simulink model "Model_AC_TES_Double_Coil"  (R2025b)
settings: Solver=VariableStepAuto  StartTime=0.0  StopTime=3600*9  RelTol=1e-3
model workspace (MAT data in the model file):
  COP = 3.9
  Delayfan = [30 1]
  P1 = 1.05
  P2 = 1.91
  P3 = 1.91
  P4 = 1.05
  Q_Cond = 4.361
  Q_Evap = 3.471
  T1 = 12
  T2 = 37.72
  T3 = 29.61
  T4 = 7.9
  T_Enviroment_C = 27.5
  T_Room_int_C = 28.6
  T_Tank_int_c = 30
  Wall_h_in = 12
  Wall_h_out = 38
  h1 = 522.3
  h2 = 528.6
  h3 = 253.4
  h4 = 253.4
  m_dot = 0.014
libraries: fl_lib x102, nesl_utility x62, SimscapeFluids_lib x31
(part 3 of 3)

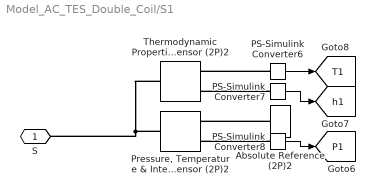
== system Model_AC_TES_Double_Coil/S1 ==
  Absolute Reference (2P)2 : fl_lib/Two-Phase Fluid/Elements/Absolute Reference (2P)
  PS-Simulink Converter6 : nesl_utility/PS-Simulink Converter  PhysicalDomain=network_engine_domain  SubClassName=ps_output  LeftPortType=input  RightPortType=output  PseudoPeriodic=off  Frequencies=[]  VectorFormat=inherit  Unit=degC  AffineConversion=on
  PS-Simulink Converter7 : nesl_utility/PS-Simulink Converter  PhysicalDomain=network_engine_domain  SubClassName=ps_output  LeftPortType=input  RightPortType=output  PseudoPeriodic=off  Frequencies=[]  VectorFormat=inherit  Unit=inherit  AffineConversion=off
  PS-Simulink Converter8 : nesl_utility/PS-Simulink Converter  PhysicalDomain=network_engine_domain  SubClassName=ps_output  LeftPortType=input  RightPortType=output  PseudoPeriodic=off  Frequencies=[]  VectorFormat=inherit  Unit=inherit  AffineConversion=off
  "Pressure, Temperature & Internal Energy Sensor (2P)2" : fl_lib/Two-Phase Fluid/Sensors/Pressure, Temperature & Internal Energy Sensor (2P)  reference=foundation.enum.MeasurementReference.difference  pressure=true  pressure_spec=foundation.enum.PressureMeasementSpec.Absolute  temperature=false  internal_energy=false
      settings: InternalSimscapePortConfiguration="{\"Bottom\":[],\"Left\":[{\"id\":\"A\",\"label\":\"A\",\"type\":\"foundation.two_phase_fluid.two_phase_fluid\"}],\"Right\":[{\"id\":\"B\",\"label\":\"B\",\"type\":\"foundation.two_phase_fluid.two_phase_fluid\"},{\"id\":\"P\",\"label\":\"P\",\"type\":\"output\"}],\"Top\":[]}"
  Thermodynamic Properties Sensor (2P)2 : fl_lib/Two-Phase Fluid/Sensors/Thermodynamic Properties Sensor (2P)  temperature=true  enthalpy=true  density=false  specific_volume=false  entropy=false
      settings: InternalSimscapePortConfiguration="{\"Bottom\":[],\"Left\":[{\"id\":\"A\",\"label\":\"A\",\"type\":\"foundation.two_phase_fluid.two_phase_fluid\"}],\"Right\":[{\"id\":\"T\",\"label\":\"T\",\"type\":\"output\"},{\"id\":\"H\",\"label\":\"h\",\"type\":\"output\"}],\"Top\":[]}"
  S : PMIOPort  Side=Left
  tag scope: P1=global, T1=global, h1=global
  wires:
  PS-Simulink Converter8/1 -> [P1]
  PS-Simulink Converter7/1 -> [h1]
  PS-Simulink Converter6/1 -> [T1]
  connections:
  Thermodynamic Properties Sensor (2P)2/LConn1 -- "Pressure, Temperature & Internal Energy Sensor (2P)2"/LConn1 -- S/RConn1
  Absolute Reference (2P)2/LConn1 -- "Pressure, Temperature & Internal Energy Sensor (2P)2"/RConn1
  PS-Simulink Converter7/LConn1 -- Thermodynamic Properties Sensor (2P)2/RConn2
  PS-Simulink Converter8/LConn1 -- "Pressure, Temperature & Internal Energy Sensor (2P)2"/RConn2
  PS-Simulink Converter6/LConn1 -- Thermodynamic Properties Sensor (2P)2/RConn1

== system Model_AC_TES_Double_Coil/S2 ==
  Absolute Reference (2P) : fl_lib/Two-Phase Fluid/Elements/Absolute Reference (2P)
  PS-Simulink Converter : nesl_utility/PS-Simulink Converter  PhysicalDomain=network_engine_domain  SubClassName=ps_output  LeftPortType=input  RightPortType=output  PseudoPeriodic=off  Frequencies=[]  VectorFormat=inherit  Unit=degC  AffineConversion=on
  PS-Simulink Converter1 : nesl_utility/PS-Simulink Converter  PhysicalDomain=network_engine_domain  SubClassName=ps_output  LeftPortType=input  RightPortType=output  PseudoPeriodic=off  Frequencies=[]  VectorFormat=inherit  Unit=inherit  AffineConversion=off
  PS-Simulink Converter2 : nesl_utility/PS-Simulink Converter  PhysicalDomain=network_engine_domain  SubClassName=ps_output  LeftPortType=input  RightPortType=output  PseudoPeriodic=off  Frequencies=[]  VectorFormat=inherit  Unit=inherit  AffineConversion=off
  "Pressure, Temperature & Internal Energy Sensor (2P)" : fl_lib/Two-Phase Fluid/Sensors/Pressure, Temperature & Internal Energy Sensor (2P)  reference=foundation.enum.MeasurementReference.difference  pressure=true  pressure_spec=foundation.enum.PressureMeasementSpec.Absolute  temperature=false  internal_energy=false
      settings: InternalSimscapePortConfiguration="{\"Bottom\":[],\"Left\":[{\"id\":\"A\",\"label\":\"A\",\"type\":\"foundation.two_phase_fluid.two_phase_fluid\"}],\"Right\":[{\"id\":\"B\",\"label\":\"B\",\"type\":\"foundation.two_phase_fluid.two_phase_fluid\"},{\"id\":\"P\",\"label\":\"P\",\"type\":\"output\"}],\"Top\":[]}"
  Thermodynamic Properties Sensor (2P) : fl_lib/Two-Phase Fluid/Sensors/Thermodynamic Properties Sensor (2P)  temperature=true  enthalpy=true  density=false  specific_volume=false  entropy=false
      settings: InternalSimscapePortConfiguration="{\"Bottom\":[],\"Left\":[{\"id\":\"A\",\"label\":\"A\",\"type\":\"foundation.two_phase_fluid.two_phase_fluid\"}],\"Right\":[{\"id\":\"T\",\"label\":\"T\",\"type\":\"output\"},{\"id\":\"H\",\"label\":\"h\",\"type\":\"output\"}],\"Top\":[]}"
  S : PMIOPort  Side=Left
  tag scope: P2=global, T2=global, h2=global
  wires:
  PS-Simulink Converter1/1 -> [h2]
  PS-Simulink Converter/1 -> [T2]
  PS-Simulink Converter2/1 -> [P2]
  connections:
  PS-Simulink Converter2/LConn1 -- "Pressure, Temperature & Internal Energy Sensor (2P)"/RConn2
  PS-Simulink Converter/LConn1 -- Thermodynamic Properties Sensor (2P)/RConn1
  Thermodynamic Properties Sensor (2P)/LConn1 -- "Pressure, Temperature & Internal Energy Sensor (2P)"/LConn1 -- S/RConn1
  Absolute Reference (2P)/LConn1 -- "Pressure, Temperature & Internal Energy Sensor (2P)"/RConn1
  PS-Simulink Converter1/LConn1 -- Thermodynamic Properties Sensor (2P)/RConn2

== system Model_AC_TES_Double_Coil/S3 ==
  Absolute Reference (2P)1 : fl_lib/Two-Phase Fluid/Elements/Absolute Reference (2P)
  PS-Simulink Converter3 : nesl_utility/PS-Simulink Converter  PhysicalDomain=network_engine_domain  SubClassName=ps_output  LeftPortType=input  RightPortType=output  PseudoPeriodic=off  Frequencies=[]  VectorFormat=inherit  Unit=degC  AffineConversion=on
  PS-Simulink Converter4 : nesl_utility/PS-Simulink Converter  PhysicalDomain=network_engine_domain  SubClassName=ps_output  LeftPortType=input  RightPortType=output  PseudoPeriodic=off  Frequencies=[]  VectorFormat=inherit  Unit=inherit  AffineConversion=off
  PS-Simulink Converter5 : nesl_utility/PS-Simulink Converter  PhysicalDomain=network_engine_domain  SubClassName=ps_output  LeftPortType=input  RightPortType=output  PseudoPeriodic=off  Frequencies=[]  VectorFormat=inherit  Unit=inherit  AffineConversion=off
  "Pressure, Temperature & Internal Energy Sensor (2P)1" : fl_lib/Two-Phase Fluid/Sensors/Pressure, Temperature & Internal Energy Sensor (2P)  reference=foundation.enum.MeasurementReference.difference  pressure=true  pressure_spec=foundation.enum.PressureMeasementSpec.Absolute  temperature=false  internal_energy=false
      settings: InternalSimscapePortConfiguration="{\"Bottom\":[],\"Left\":[{\"id\":\"A\",\"label\":\"A\",\"type\":\"foundation.two_phase_fluid.two_phase_fluid\"}],\"Right\":[{\"id\":\"B\",\"label\":\"B\",\"type\":\"foundation.two_phase_fluid.two_phase_fluid\"},{\"id\":\"P\",\"label\":\"P\",\"type\":\"output\"}],\"Top\":[]}"
  Thermodynamic Properties Sensor (2P)1 : fl_lib/Two-Phase Fluid/Sensors/Thermodynamic Properties Sensor (2P)  temperature=true  enthalpy=true  density=false  specific_volume=false  entropy=false
      settings: InternalSimscapePortConfiguration="{\"Bottom\":[],\"Left\":[{\"id\":\"A\",\"label\":\"A\",\"type\":\"foundation.two_phase_fluid.two_phase_fluid\"}],\"Right\":[{\"id\":\"T\",\"label\":\"T\",\"type\":\"output\"},{\"id\":\"H\",\"label\":\"h\",\"type\":\"output\"}],\"Top\":[]}"
  S : PMIOPort  Side=Left
  tag scope: P3=global, T3=global, h3=global
  wires:
  PS-Simulink Converter4/1 -> [h3]
  PS-Simulink Converter3/1 -> [T3]
  PS-Simulink Converter5/1 -> [P3]
  connections:
  Absolute Reference (2P)1/LConn1 -- "Pressure, Temperature & Internal Energy Sensor (2P)1"/RConn1
  PS-Simulink Converter3/LConn1 -- Thermodynamic Properties Sensor (2P)1/RConn1
  PS-Simulink Converter4/LConn1 -- Thermodynamic Properties Sensor (2P)1/RConn2
  Thermodynamic Properties Sensor (2P)1/LConn1 -- "Pressure, Temperature & Internal Energy Sensor (2P)1"/LConn1 -- S/RConn1
  PS-Simulink Converter5/LConn1 -- "Pressure, Temperature & Internal Energy Sensor (2P)1"/RConn2

== system Model_AC_TES_Double_Coil/S4 ==
  Absolute Reference (2P)2 : fl_lib/Two-Phase Fluid/Elements/Absolute Reference (2P)
  PS-Simulink Converter6 : nesl_utility/PS-Simulink Converter  PhysicalDomain=network_engine_domain  SubClassName=ps_output  LeftPortType=input  RightPortType=output  PseudoPeriodic=off  Frequencies=[]  VectorFormat=inherit  Unit=degC  AffineConversion=on
  PS-Simulink Converter7 : nesl_utility/PS-Simulink Converter  PhysicalDomain=network_engine_domain  SubClassName=ps_output  LeftPortType=input  RightPortType=output  PseudoPeriodic=off  Frequencies=[]  VectorFormat=inherit  Unit=inherit  AffineConversion=off
  PS-Simulink Converter8 : nesl_utility/PS-Simulink Converter  PhysicalDomain=network_engine_domain  SubClassName=ps_output  LeftPortType=input  RightPortType=output  PseudoPeriodic=off  Frequencies=[]  VectorFormat=inherit  Unit=inherit  AffineConversion=off
  "Pressure, Temperature & Internal Energy Sensor (2P)2" : fl_lib/Two-Phase Fluid/Sensors/Pressure, Temperature & Internal Energy Sensor (2P)  reference=foundation.enum.MeasurementReference.difference  pressure=true  pressure_spec=foundation.enum.PressureMeasementSpec.Absolute  temperature=false  internal_energy=false
      settings: InternalSimscapePortConfiguration="{\"Bottom\":[],\"Left\":[{\"id\":\"A\",\"label\":\"A\",\"type\":\"foundation.two_phase_fluid.two_phase_fluid\"}],\"Right\":[{\"id\":\"B\",\"label\":\"B\",\"type\":\"foundation.two_phase_fluid.two_phase_fluid\"},{\"id\":\"P\",\"label\":\"P\",\"type\":\"output\"}],\"Top\":[]}"
  Thermodynamic Properties Sensor (2P)2 : fl_lib/Two-Phase Fluid/Sensors/Thermodynamic Properties Sensor (2P)  temperature=true  enthalpy=true  density=false  specific_volume=false  entropy=false
      settings: InternalSimscapePortConfiguration="{\"Bottom\":[],\"Left\":[{\"id\":\"A\",\"label\":\"A\",\"type\":\"foundation.two_phase_fluid.two_phase_fluid\"}],\"Right\":[{\"id\":\"T\",\"label\":\"T\",\"type\":\"output\"},{\"id\":\"H\",\"label\":\"h\",\"type\":\"output\"}],\"Top\":[]}"
  S : PMIOPort  Side=Left
  tag scope: P4=global, T4=global, h4=global
  wires:
  PS-Simulink Converter8/1 -> [P4]
  PS-Simulink Converter7/1 -> [h4]
  PS-Simulink Converter6/1 -> [T4]
  connections:
  Thermodynamic Properties Sensor (2P)2/LConn1 -- "Pressure, Temperature & Internal Energy Sensor (2P)2"/LConn1 -- S/RConn1
  Absolute Reference (2P)2/LConn1 -- "Pressure, Temperature & Internal Energy Sensor (2P)2"/RConn1
  PS-Simulink Converter7/LConn1 -- Thermodynamic Properties Sensor (2P)2/RConn2
  PS-Simulink Converter8/LConn1 -- "Pressure, Temperature & Internal Energy Sensor (2P)2"/RConn2
  PS-Simulink Converter6/LConn1 -- Thermodynamic Properties Sensor (2P)2/RConn1

== system Model_AC_TES_Double_Coil/S5 ==
  Absolute Reference (2P)2 : fl_lib/Two-Phase Fluid/Elements/Absolute Reference (2P)
  PS-Simulink Converter6 : nesl_utility/PS-Simulink Converter  PhysicalDomain=network_engine_domain  SubClassName=ps_output  LeftPortType=input  RightPortType=output  PseudoPeriodic=off  Frequencies=[]  VectorFormat=inherit  Unit=degC  AffineConversion=on
  PS-Simulink Converter7 : nesl_utility/PS-Simulink Converter  PhysicalDomain=network_engine_domain  SubClassName=ps_output  LeftPortType=input  RightPortType=output  PseudoPeriodic=off  Frequencies=[]  VectorFormat=inherit  Unit=inherit  AffineConversion=off
  PS-Simulink Converter8 : nesl_utility/PS-Simulink Converter  PhysicalDomain=network_engine_domain  SubClassName=ps_output  LeftPortType=input  RightPortType=output  PseudoPeriodic=off  Frequencies=[]  VectorFormat=inherit  Unit=inherit  AffineConversion=off
  "Pressure, Temperature & Internal Energy Sensor (2P)2" : fl_lib/Two-Phase Fluid/Sensors/Pressure, Temperature & Internal Energy Sensor (2P)  reference=foundation.enum.MeasurementReference.difference  pressure=true  pressure_spec=foundation.enum.PressureMeasementSpec.Absolute  temperature=false  internal_energy=false
      settings: InternalSimscapePortConfiguration="{\"Bottom\":[],\"Left\":[{\"id\":\"A\",\"label\":\"A\",\"type\":\"foundation.two_phase_fluid.two_phase_fluid\"}],\"Right\":[{\"id\":\"B\",\"label\":\"B\",\"type\":\"foundation.two_phase_fluid.two_phase_fluid\"},{\"id\":\"P\",\"label\":\"P\",\"type\":\"output\"}],\"Top\":[]}"
  Thermodynamic Properties Sensor (2P)2 : fl_lib/Two-Phase Fluid/Sensors/Thermodynamic Properties Sensor (2P)  temperature=true  enthalpy=true  density=false  specific_volume=false  entropy=false
      settings: InternalSimscapePortConfiguration="{\"Bottom\":[],\"Left\":[{\"id\":\"A\",\"label\":\"A\",\"type\":\"foundation.two_phase_fluid.two_phase_fluid\"}],\"Right\":[{\"id\":\"T\",\"label\":\"T\",\"type\":\"output\"},{\"id\":\"H\",\"label\":\"h\",\"type\":\"output\"}],\"Top\":[]}"
  S : PMIOPort  Side=Left
  tag scope: P5=global, T5=global, h5=global
  wires:
  PS-Simulink Converter8/1 -> [P5]
  PS-Simulink Converter7/1 -> [h5]
  PS-Simulink Converter6/1 -> [T5]
  connections:
  Thermodynamic Properties Sensor (2P)2/LConn1 -- "Pressure, Temperature & Internal Energy Sensor (2P)2"/LConn1 -- S/RConn1
  Absolute Reference (2P)2/LConn1 -- "Pressure, Temperature & Internal Energy Sensor (2P)2"/RConn1
  PS-Simulink Converter7/LConn1 -- Thermodynamic Properties Sensor (2P)2/RConn2
  PS-Simulink Converter8/LConn1 -- "Pressure, Temperature & Internal Energy Sensor (2P)2"/RConn2
  PS-Simulink Converter6/LConn1 -- Thermodynamic Properties Sensor (2P)2/RConn1

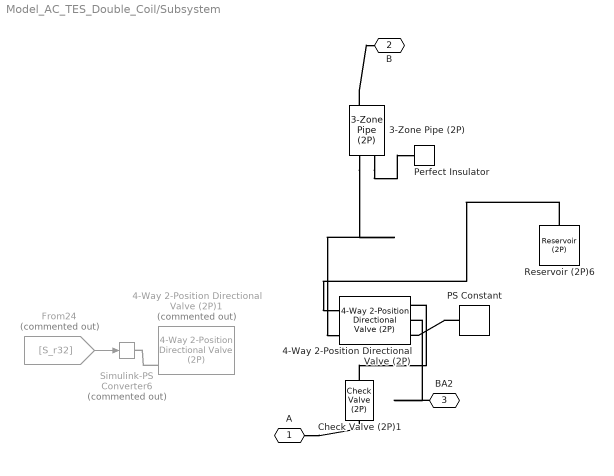
== system Model_AC_TES_Double_Coil/Subsystem ==
  3-Zone Pipe (2P) : SimscapeFluids_lib/Two-Phase Fluid/Pipes & Fittings/3-Zone Pipe (2P)  length=0.1 m  area=0.01 m^2  Dh=0.1 m  elevation_gain=0 m  g=9.81 m/s^2  length_add=0.1 m  roughness=15e-6 m  Re_lam=2000  Re_tur=4000  shape_factor=64  hc_ext=100 W/(K*m^2)  wall_thickness=0 m  k_wall=390 W/(K*m)  c_wall=390 J/(K*kg)  rho_wall=9e3 kg/m^3  fin_ratio_ext=0  eta_fin_ext=0.5  fin_ratio_int=0  eta_fin_int=0.5  heat_coeff_spec=fluids.two_phase_fluid.pipes_fittings.enum.HeatCoeffSpec.GnielinskiCavalliniZecchin  colburn_coeff_liq=[.023, .8, .33]  colburn_coeff_mix=[.05, .8, .33]  colburn_coeff_vap=[.023, .8, .33]  Nu_lam=3.66  energy_spec=foundation.enum.energy_spec.temperature  p_init=P1 MPa  T_init=12 degC  x_init=0.5  alpha_init=0.5  h_init=1500 kJ/kg  u_init=1500 kJ/kg
      settings: InternalSimscapePortConfiguration="{\"Bottom\":[],\"Left\":[{\"id\":\"A\",\"label\":\"A\",\"type\":\"foundation.two_phase_fluid.two_phase_fluid\"},{\"id\":\"H\",\"label\":\"H\",\"type\":\"foundation.thermal.thermal\"}],\"Right\":[{\"id\":\"B\",\"label\":\"B\",\"type\":\"foundation.two_phase_fluid.two_phase_fluid\"},{\"id\":\"Z\",\"label\":\"Z\",\"type\":\"output\"}],\"Top\":[]}"
  4-Way 2-Position Directional Valve (2P) : SimscapeFluids_lib/Two-Phase Fluid/Valves & Orifices/Directional Control Valves/4-Way 2-Position Directional Valve (2P)  open_orifices_pos=fluids.two_phase_fluid.valves_orifices.directional_control_valves.enum.OpenOrifices4Way2Position.PA_PB  open_orifices_neg=fluids.two_phase_fluid.valves_orifices.directional_control_valves.enum.OpenOrifices4Way2Position.PB_AT  area_spec=fluids.two_phase_fluid.valves_orifices.directional_control_valves.enum.AreaSpec.Identical  liquid_valve_parameterization=fluids.two_phase_fluid.valves_orifices.directional_control_valves.enum.LiquidOrificeParameterization.LinearArea  del_S_max=0.11 m  mdot_nominal_max=0.1 kg/s  delta_p_nominal_max=0.001 MPa  energy_spec=foundation.enum.energy_spec.temperature  p_inlet=0.101325 MPa  T_inlet=293.15 K  x_inlet=0  alpha_inlet=0  h_inlet=400 kJ/kg  u_inlet=400 kJ/kg  valve_area_max=0.1 m^2  del_S_TLU=[0, .00125, .0025, .00375, .005] m  valve_area_TLU=[1e-10, 1e-05, 4e-05, 6e-05, .0001] m^2  Cd=0.64  pressure_recovery=false  leakage_fraction=1e-6  smoothing_factor=0.01  B_lam=0.999  tau_x=0.1 s  area=0.11 m^2  S_max_PA=0.1 m  del_S_max_PA=0.005 m  mdot_nominal_max_PA=0.1 kg/s  delta_p_nominal_max_PA=0.001 MPa  energy_spec_PA=foundation.enum.energy_spec.temperature  p_inlet_PA=0.101325 MPa  T_inlet_PA=293.15 K  x_inlet_PA=0  alpha_inlet_PA=0  h_inlet_PA=400 kJ/kg  u_inlet_PA=400 kJ/kg  valve_area_max_PA=1e-4 m^2  del_S_TLU_PA=[0, .00125, .0025, .00375, .005] m  valve_area_TLU_PA=[1e-10, 1e-05, 4e-05, 6e-05, .0001] m^2  mdot_nominal_const_PA=0.1 kg/s  delta_p_nominal_const_PA=0.001 MPa  valve_area_const_PA=1e-4 m^2  S_max_PB=-5e-3 m  del_S_max_PB=0.005 m  mdot_nominal_max_PB=0.1 kg/s  delta_p_nominal_max_PB=0.001 MPa  energy_spec_PB=foundation.enum.energy_spec.temperature  p_inlet_PB=0.101325 MPa  T_inlet_PB=293.15 K  x_inlet_PB=0  alpha_inlet_PB=0  h_inlet_PB=400 kJ/kg  u_inlet_PB=400 kJ/kg  valve_area_max_PB=1e-4 m^2  del_S_TLU_PB=[0, .00125, .0025, .00375, .005] m  valve_area_TLU_PB=[1e-10, 1e-05, 4e-05, 6e-05, .0001] m^2  mdot_nominal_const_PB=0.1 kg/s  delta_p_nominal_const_PB=0.001 MPa  valve_area_const_PB=1e-4 m^2  S_max_AT=-0.1 m  del_S_max_AT=0.005 m  mdot_nominal_max_AT=0.1 kg/s  delta_p_nominal_max_AT=0.001 MPa  energy_spec_AT=foundation.enum.energy_spec.temperature  p_inlet_AT=0.101325 MPa  T_inlet_AT=293.15 K  x_inlet_AT=0  alpha_inlet_AT=0  h_inlet_AT=400 kJ/kg  u_inlet_AT=400 kJ/kg  valve_area_max_AT=1e-4 m^2  del_S_TLU_AT=[0, .00125, .0025, .00375, .005] m  valve_area_TLU_AT=[1e-10, 1e-05, 4e-05, 6e-05, .0001] m^2  mdot_nominal_const_AT=0.1 kg/s  delta_p_nominal_const_AT=0.001 MPa  valve_area_const_AT=1e-4 m^2  S_max_BT=5e-3 m  del_S_max_BT=0.005 m  mdot_nominal_max_BT=0.1 kg/s  delta_p_nominal_max_BT=0.001 MPa  energy_spec_BT=foundation.enum.energy_spec.temperature  p_inlet_BT=0.101325 MPa  T_inlet_BT=293.15 K  x_inlet_BT=0  alpha_inlet_BT=0  h_inlet_BT=400 kJ/kg  u_inlet_BT=400 kJ/kg  valve_area_max_BT=1e-4 m^2  del_S_TLU_BT=[0, .00125, .0025, .00375, .005] m  valve_area_TLU_BT=[1e-10, 1e-05, 4e-05, 6e-05, .0001] m^2  mdot_nominal_const_BT=0.1 kg/s  delta_p_nominal_const_BT=0.001 MPa  valve_area_const_BT=1e-4 m^2  vapor_valve_parameterization=fluids.two_phase_fluid.valves_orifices.enum.VaporOrificeParameterization.Cv  opening_characteristic=fluids.two_phase_fluid.valves_orifices.enum.OpeningCharacteristics.Linear  Cv_max=4  del_S_Cv_TLU=[0, .001, .002, .003, .004, .005] m  Cv_TLU=[1e-06, .8, 1.6, 2.4, 3.2, 4]  xT_Cv=0.7  Kv_max=3.6  del_S_Kv_TLU=[0, .001, .002, .003, .004, .005] m  Kv_TLU=[1e-06, .72, 1.44, 2.16, 2.88, 3.6]  xT_Kv=0.7  orifice_area_max=1e-4 m^2  del_S_orifice_area_TLU=[0, .001, .002, .003, .004, .005] m  orifice_area_TLU=[1e-10, 2e-05, 4e-05, 6e-05, 8e-05, .0001] m^2  Cv_const_PA=4  Cv_max_PA=4  del_S_Cv_TLU_PA=[0, .001, .002, .003, .004, .005] m  Cv_TLU_PA=[1e-06, .8, 1.6, 2.4, 3.2, 4]  xT_Cv_PA=0.7  Kv_const_PA=3.6  Kv_max_PA=3.6  del_S_Kv_TLU_PA=[0, .001, .002, .003, .004, .005] m  Kv_TLU_PA=[1e-06, .72, 1.44, 2.16, 2.88, 3.6]  xT_Kv_PA=0.7  orifice_area_const_PA=1e-4 m^2  orifice_area_max_PA=1e-4 m^2  del_S_orifice_area_TLU_PA=[0, .001, .002, .003, .004, .005] m  orifice_area_TLU_PA=[1e-10, 2e-05, 4e-05, 6e-05, 8e-05, .0001] m^2  Cv_const_PB=4  Cv_max_PB=4  del_S_Cv_TLU_PB=[0, .001, .002, .003, .004, .005] m  Cv_TLU_PB=[1e-06, .8, 1.6, 2.4, 3.2, 4]  xT_Cv_PB=0.7  Kv_const_PB=3.6  Kv_max_PB=3.6  del_S_Kv_TLU_PB=[0, .001, .002, .003, .004, .005] m  Kv_TLU_PB=[1e-06, .72, 1.44, 2.16, 2.88, 3.6]  xT_Kv_PB=0.7  orifice_area_const_PB=1e-4 m^2  orifice_area_max_PB=1e-4 m^2  del_S_orifice_area_TLU_PB=[0, .001, .002, .003, .004, .005] m  orifice_area_TLU_PB=[1e-10, 2e-05, 4e-05, 6e-05, 8e-05, .0001] m^2  Cv_const_AT=4  Cv_max_AT=4  del_S_Cv_TLU_AT=[0, .001, .002, .003, .004, .005] m  Cv_TLU_AT=[1e-06, .8, 1.6, 2.4, 3.2, 4]  xT_Cv_AT=0.7  Kv_const_AT=3.6  Kv_max_AT=3.6  del_S_Kv_TLU_AT=[0, .001, .002, .003, .004, .005] m  Kv_TLU_AT=[1e-06, .72, 1.44, 2.16, 2.88, 3.6]  xT_Kv_AT=0.7  orifice_area_const_AT=1e-4 m^2  orifice_area_max_AT=1e-4 m^2  del_S_orifice_area_TLU_AT=[0, .001, .002, .003, .004, .005] m  orifice_area_TLU_AT=[1e-10, 2e-05, 4e-05, 6e-05, 8e-05, .0001] m^2  Cv_const_BT=4  Cv_max_BT=4  del_S_Cv_TLU_BT=[0, .001, .002, .003, .004, .005] m  Cv_TLU_BT=[1e-06, .8, 1.6, 2.4, 3.2, 4]  xT_Cv_BT=0.7  Kv_const_BT=3.6  Kv_max_BT=3.6  del_S_Kv_TLU_BT=[0, .001, .002, .003, .004, .005] m  Kv_TLU_BT=[1e-06, .72, 1.44, 2.16, 2.88, 3.6]  xT_Kv_BT=0.7  orifice_area_const_BT=1e-4 m^2  orifice_area_max_BT=1e-4 m^2  del_S_orifice_area_TLU_BT=[0, .001, .002, .003, .004, .005] m  orifice_area_TLU_BT=[1e-10, 2e-05, 4e-05, 6e-05, 8e-05, .0001] m^2
      settings: InternalSimscapePortConfiguration="{\"Bottom\":[{\"id\":\"P\",\"label\":\"P\",\"type\":\"foundation.two_phase_fluid.two_phase_fluid\"},{\"id\":\"T\",\"label\":\"T\",\"type\":\"foundation.two_phase_fluid.two_phase_fluid\"}],\"Left\":[{\"id\":\"S\",\"label\":\"S\",\"type\":\"input\"}],\"Right\":[],\"Top\":[{\"id\":\"A\",\"label\":\"A\",\"type\":\"foundation.two_phase_fluid.two_phase_fluid\"},{\"id\":\"B\",\"label\":\"B\",\"type\":\"foundation.two_phase_fluid.two_phase_fluid\"}]}"
  4-Way 2-Position Directional Valve (2P)1 : SimscapeFluids_lib/Two-Phase Fluid/Valves & Orifices/Directional Control Valves/4-Way 2-Position Directional Valve (2P)  Commented=on  open_orifices_pos=fluids.two_phase_fluid.valves_orifices.directional_control_valves.enum.OpenOrifices4Way2Position.PA_BT  open_orifices_neg=fluids.two_phase_fluid.valves_orifices.directional_control_valves.enum.OpenOrifices4Way2Position.PA_PB  area_spec=fluids.two_phase_fluid.valves_orifices.directional_control_valves.enum.AreaSpec.Identical  liquid_valve_parameterization=fluids.two_phase_fluid.valves_orifices.directional_control_valves.enum.LiquidOrificeParameterization.LinearArea  del_S_max=0.005 m  mdot_nominal_max=0.1 kg/s  delta_p_nominal_max=0.001 MPa  energy_spec=foundation.enum.energy_spec.temperature  p_inlet=0.101325 MPa  T_inlet=293.15 K  x_inlet=0  alpha_inlet=0  h_inlet=400 kJ/kg  u_inlet=400 kJ/kg  valve_area_max=1e-4 m^2  del_S_TLU=[0, .00125, .0025, .00375, .005] m  valve_area_TLU=[1e-10, 1e-05, 4e-05, 6e-05, .0001] m^2  Cd=0.64  pressure_recovery=false  leakage_fraction=1e-6  smoothing_factor=0.01  B_lam=0.999  tau_x=0.1 s  area=0.01 m^2  S_max_PA=0.01 m  del_S_max_PA=0.005 m  mdot_nominal_max_PA=0.1 kg/s  delta_p_nominal_max_PA=0.001 MPa  energy_spec_PA=foundation.enum.energy_spec.temperature  p_inlet_PA=0.101325 MPa  T_inlet_PA=293.15 K  x_inlet_PA=0  alpha_inlet_PA=0  h_inlet_PA=400 kJ/kg  u_inlet_PA=400 kJ/kg  valve_area_max_PA=1e-4 m^2  del_S_TLU_PA=[0, .00125, .0025, .00375, .005] m  valve_area_TLU_PA=[1e-10, 1e-05, 4e-05, 6e-05, .0001] m^2  mdot_nominal_const_PA=0.1 kg/s  delta_p_nominal_const_PA=0.001 MPa  valve_area_const_PA=1e-4 m^2  S_max_PB=0.01 m  del_S_max_PB=0.005 m  mdot_nominal_max_PB=0.1 kg/s  delta_p_nominal_max_PB=0.001 MPa  energy_spec_PB=foundation.enum.energy_spec.temperature  p_inlet_PB=0.101325 MPa  T_inlet_PB=293.15 K  x_inlet_PB=0  alpha_inlet_PB=0  h_inlet_PB=400 kJ/kg  u_inlet_PB=400 kJ/kg  valve_area_max_PB=1e-4 m^2  del_S_TLU_PB=[0, .00125, .0025, .00375, .005] m  valve_area_TLU_PB=[1e-10, 1e-05, 4e-05, 6e-05, .0001] m^2  mdot_nominal_const_PB=0.1 kg/s  delta_p_nominal_const_PB=0.001 MPa  valve_area_const_PB=1e-4 m^2  S_max_AT=-5e-3 m  del_S_max_AT=0.005 m  mdot_nominal_max_AT=0.1 kg/s  delta_p_nominal_max_AT=0.001 MPa  energy_spec_AT=foundation.enum.energy_spec.temperature  p_inlet_AT=0.101325 MPa  T_inlet_AT=293.15 K  x_inlet_AT=0  alpha_inlet_AT=0  h_inlet_AT=400 kJ/kg  u_inlet_AT=400 kJ/kg  valve_area_max_AT=1e-4 m^2  del_S_TLU_AT=[0, .00125, .0025, .00375, .005] m  valve_area_TLU_AT=[1e-10, 1e-05, 4e-05, 6e-05, .0001] m^2  mdot_nominal_const_AT=0.1 kg/s  delta_p_nominal_const_AT=0.001 MPa  valve_area_const_AT=1e-4 m^2  S_max_BT=5e-3 m  del_S_max_BT=0.005 m  mdot_nominal_max_BT=0.1 kg/s  delta_p_nominal_max_BT=0.001 MPa  energy_spec_BT=foundation.enum.energy_spec.temperature  p_inlet_BT=0.101325 MPa  T_inlet_BT=293.15 K  x_inlet_BT=0  alpha_inlet_BT=0  h_inlet_BT=400 kJ/kg  u_inlet_BT=400 kJ/kg  valve_area_max_BT=1e-4 m^2  del_S_TLU_BT=[0, .00125, .0025, .00375, .005] m  valve_area_TLU_BT=[1e-10, 1e-05, 4e-05, 6e-05, .0001] m^2  mdot_nominal_const_BT=0.1 kg/s  delta_p_nominal_const_BT=0.001 MPa  valve_area_const_BT=1e-4 m^2  vapor_valve_parameterization=fluids.two_phase_fluid.valves_orifices.enum.VaporOrificeParameterization.Cv  opening_characteristic=fluids.two_phase_fluid.valves_orifices.enum.OpeningCharacteristics.Linear  Cv_max=4  del_S_Cv_TLU=[0, .001, .002, .003, .004, .005] m  Cv_TLU=[1e-06, .8, 1.6, 2.4, 3.2, 4]  xT_Cv=0.7  Kv_max=3.6  del_S_Kv_TLU=[0, .001, .002, .003, .004, .005] m  Kv_TLU=[1e-06, .72, 1.44, 2.16, 2.88, 3.6]  xT_Kv=0.7  orifice_area_max=1e-4 m^2  del_S_orifice_area_TLU=[0, .001, .002, .003, .004, .005] m  orifice_area_TLU=[1e-10, 2e-05, 4e-05, 6e-05, 8e-05, .0001] m^2  Cv_const_PA=4  Cv_max_PA=4  del_S_Cv_TLU_PA=[0, .001, .002, .003, .004, .005] m  Cv_TLU_PA=[1e-06, .8, 1.6, 2.4, 3.2, 4]  xT_Cv_PA=0.7  Kv_const_PA=3.6  Kv_max_PA=3.6  del_S_Kv_TLU_PA=[0, .001, .002, .003, .004, .005] m  Kv_TLU_PA=[1e-06, .72, 1.44, 2.16, 2.88, 3.6]  xT_Kv_PA=0.7  orifice_area_const_PA=1e-4 m^2  orifice_area_max_PA=1e-4 m^2  del_S_orifice_area_TLU_PA=[0, .001, .002, .003, .004, .005] m  orifice_area_TLU_PA=[1e-10, 2e-05, 4e-05, 6e-05, 8e-05, .0001] m^2  Cv_const_PB=4  Cv_max_PB=4  del_S_Cv_TLU_PB=[0, .001, .002, .003, .004, .005] m  Cv_TLU_PB=[1e-06, .8, 1.6, 2.4, 3.2, 4]  xT_Cv_PB=0.7  Kv_const_PB=3.6  Kv_max_PB=3.6  del_S_Kv_TLU_PB=[0, .001, .002, .003, .004, .005] m  Kv_TLU_PB=[1e-06, .72, 1.44, 2.16, 2.88, 3.6]  xT_Kv_PB=0.7  orifice_area_const_PB=1e-4 m^2  orifice_area_max_PB=1e-4 m^2  del_S_orifice_area_TLU_PB=[0, .001, .002, .003, .004, .005] m  orifice_area_TLU_PB=[1e-10, 2e-05, 4e-05, 6e-05, 8e-05, .0001] m^2  Cv_const_AT=4  Cv_max_AT=4  del_S_Cv_TLU_AT=[0, .001, .002, .003, .004, .005] m  Cv_TLU_AT=[1e-06, .8, 1.6, 2.4, 3.2, 4]  xT_Cv_AT=0.7  Kv_const_AT=3.6  Kv_max_AT=3.6  del_S_Kv_TLU_AT=[0, .001, .002, .003, .004, .005] m  Kv_TLU_AT=[1e-06, .72, 1.44, 2.16, 2.88, 3.6]  xT_Kv_AT=0.7  orifice_area_const_AT=1e-4 m^2  orifice_area_max_AT=1e-4 m^2  del_S_orifice_area_TLU_AT=[0, .001, .002, .003, .004, .005] m  orifice_area_TLU_AT=[1e-10, 2e-05, 4e-05, 6e-05, 8e-05, .0001] m^2  Cv_const_BT=4  Cv_max_BT=4  del_S_Cv_TLU_BT=[0, .001, .002, .003, .004, .005] m  Cv_TLU_BT=[1e-06, .8, 1.6, 2.4, 3.2, 4]  xT_Cv_BT=0.7  Kv_const_BT=3.6  Kv_max_BT=3.6  del_S_Kv_TLU_BT=[0, .001, .002, .003, .004, .005] m  Kv_TLU_BT=[1e-06, .72, 1.44, 2.16, 2.88, 3.6]  xT_Kv_BT=0.7  orifice_area_const_BT=1e-4 m^2  orifice_area_max_BT=1e-4 m^2  del_S_orifice_area_TLU_BT=[0, .001, .002, .003, .004, .005] m  orifice_area_TLU_BT=[1e-10, 2e-05, 4e-05, 6e-05, 8e-05, .0001] m^2
      settings: InternalSimscapePortConfiguration="{\"Bottom\":[{\"id\":\"P\",\"label\":\"P\",\"type\":\"foundation.two_phase_fluid.two_phase_fluid\"},{\"id\":\"T\",\"label\":\"T\",\"type\":\"foundation.two_phase_fluid.two_phase_fluid\"}],\"Left\":[{\"id\":\"S\",\"label\":\"S\",\"type\":\"input\"}],\"Right\":[],\"Top\":[{\"id\":\"A\",\"label\":\"A\",\"type\":\"foundation.two_phase_fluid.two_phase_fluid\"},{\"id\":\"B\",\"label\":\"B\",\"type\":\"foundation.two_phase_fluid.two_phase_fluid\"}]}"
  Check Valve (2P)1 : SimscapeFluids_lib/Two-Phase Fluid/Valves & Orifices/Directional Control Valves/Check Valve (2P)  liquid_valve_parameterization=fluids.two_phase_fluid.valves_orifices.enum.LiquidPressureValveParameterization.LinearArea  opening_pressure_spec=fluids.two_phase_fluid.valves_orifices.enum.PressureControlSpec.PressureDifferential  p_crack_differential=0.01 MPa  p_crack_gauge=0.1 MPa  p_max_differential=0.1 MPa  p_max_gauge=0.2 MPa  mdot_nominal_max=0.1 kg/s  delta_p_nominal_max=0.001 MPa  valve_area_max=1e-4 m^2  p_diff_TLU=[0.2 : 0.2 : 1.2] MPa  p_gauge_TLU=[0.2 : 0.2 : 1.2] MPa  valve_area_TLU=[1e-10, 2e-06, 4e-06, 6e-06, 8e-06, 1e-05] m^2  energy_spec=foundation.enum.energy_spec.temperature  p_inlet=0.101325 MPa  T_inlet=293.15 K  x_inlet=0  alpha_inlet=0  h_inlet=400 kJ/kg  u_inlet=400 kJ/kg  Cd=0.64  pressure_recovery=false  leakage_fraction=1e-6  smoothing_factor=0.01  B_lam=0.999  tau_x=0.1 s  area=0.01 m^2  vapor_valve_parameterization=fluids.two_phase_fluid.valves_orifices.enum.VaporOrificeParameterization.Cv  opening_characteristic=fluids.two_phase_fluid.valves_orifices.enum.OpeningCharacteristics.Linear  Cv_max=4  p_diff_Cv_TLU=0.2 : 0.2 : 1.2 MPa  p_gauge_Cv_TLU=0.2 : 0.2 : 1.2 MPa  Cv_TLU=[1e-06, .8, 1.6, 2.4, 3.2, 4]  xT_Cv=0.7  Kv_max=3.6  p_diff_Kv_TLU=0.2 : 0.2 : 1.2 MPa  p_gauge_Kv_TLU=0.2 : 0.2 : 1.2 MPa  Kv_TLU=[1e-06, .72, 1.44, 2.16, 2.88, 3.6]  xT_Kv=0.7  orifice_area_max=1e-4 m^2  p_diff_orifice_area_TLU=0.2 : 0.2 : 1.2 MPa  p_gauge_orifice_area_TLU=0.2 : 0.2 : 1.2 MPa  orifice_area_TLU=[1e-10, 2e-05, 4e-05, 6e-05, 8e-05, .0001] m^2
      settings: InternalSimscapePortConfiguration="{\"Bottom\":[],\"Left\":[{\"id\":\"A\",\"label\":\"A\",\"type\":\"foundation.two_phase_fluid.two_phase_fluid\"}],\"Right\":[{\"id\":\"B\",\"label\":\"B\",\"type\":\"foundation.two_phase_fluid.two_phase_fluid\"}],\"Top\":[]}"
  From24 : From  Commented=on  GotoTag=S_r32  TagVisibility=global
  PS Constant : fl_lib/Physical Signals/Sources/PS Constant  constant=1
  Perfect Insulator : fl_lib/Thermal/Thermal Elements/Perfect Insulator  T_specify=off  T_priority=None  T=293.15 K  T_nominal_specify=off  T_nominal_value=1  T_nominal_unit=K
  Reservoir (2P)6 : fl_lib/Two-Phase Fluid/Elements/Reservoir (2P)  pressure_spec=foundation.enum.ReservoirPressureSpec2P.Specified  reservoir_pressure=0.8 MPa  reservoir_condensing_temperature=373.15 K  reservoir_evaporating_temperature=373.15 K  energy_spec=foundation.enum.ReservoirEnergySpec2P.Temperature  reservoir_temperature=8 degC  reservoir_quality=0.5  reservoir_void_fraction=0.5  reservoir_enthalpy=1500 kJ/kg  reservoir_internal_energy=1500 kJ/kg  reservoir_subcooling=5 deltaK  reservoir_superheating=5 deltaK  area_A=0.01 m^2
  Simulink-PS Converter6 : nesl_utility/Simulink-PS Converter  Commented=on  PhysicalDomain=network_engine_domain  SubClassName=ps_input  LeftPortType=input  RightPortType=output  PseudoPeriodic=off  Frequencies=[]  NoiseDistribution=none  NoiseParameters=[]  Unit=1  AffineConversion=off  FilteringAndDerivatives=provide  SimscapeFilterOrder=1  InputFilterTimeConstant=0.001  UdotUserProvided=0
  A : PMIOPort  Side=Left
  B : PMIOPort  Port=2  Side=Left
  BA2 : PMIOPort  Port=3  Side=Right
  wires:
  From24/1 -> Simulink-PS Converter6/1
  connections:
  4-Way 2-Position Directional Valve (2P)1/LConn1 -- Simulink-PS Converter6/RConn1
  BA2/RConn1 -- 4-Way 2-Position Directional Valve (2P)/LConn2
  3-Zone Pipe (2P)/LConn2 -- Perfect Insulator/LConn1
  Check Valve (2P)1/RConn1 -- 4-Way 2-Position Directional Valve (2P)/LConn3
  3-Zone Pipe (2P)/RConn1 -- B/RConn1
  3-Zone Pipe (2P)/LConn1 -- 4-Way 2-Position Directional Valve (2P)/RConn1
  PS Constant/RConn1 -- 4-Way 2-Position Directional Valve (2P)/LConn1
  Reservoir (2P)6/LConn1 -- 4-Way 2-Position Directional Valve (2P)/RConn2
  A/RConn1 -- Check Valve (2P)1/LConn1

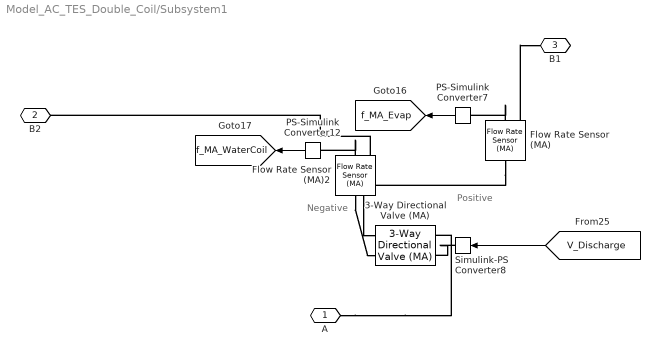
== system Model_AC_TES_Double_Coil/Subsystem1 ==
  note: Negative
  note: Positive
  3-Way Directional Valve (MA) : SimscapeFluids_lib/Moist Air/Valves & Orifices/Directional Control Valves/3-Way Directional Valve (MA)  open_orifices_pos=fluids.moist_air.valves_orifices.directional_control_valves.enum.OpenOrifices3Way.AT  open_orifices_neg=fluids.moist_air.valves_orifices.directional_control_valves.enum.OpenOrifices3Way.PA  area_spec=fluids.moist_air.valves_orifices.directional_control_valves.enum.AreaSpec.Identical  valve_parameterization=fluids.moist_air.valves_orifices.enum.OrificeParameterization.Area  opening_characteristic=fluids.moist_air.valves_orifices.enum.OpeningCharacteristics.Linear  del_S_max=0.01 m  Cv_max=4  del_S_Cv_TLU=[0, .003, .006, .009, .012, .015] m  Cv_TLU=[1e-06, .8, 1.6, 2.4, 3.2, 4]  xT_Cv=0.7  Kv_max=3.6  del_S_Kv_TLU=[0, .003, .006, .009, .012, .015] m  Kv_TLU=[1e-06, .72, 1.44, 2.16, 2.88, 3.6]  xT_Kv=0.7  C_max=12 l/(bar*s)  B_crit_linear=0.3  del_S_C_TLU=[0, .003, .006, .009, .012, .015] m  C_TLU=[1e-05, 2.4, 4.8, 7.2, 9.6, 12] l/(bar*s)  B_crit_TLU=0.3 * ones(1, 6)  m=0.5  T_ref_C=293.15 K  rho_ref_C=1.185 kg/m^3  orifice_area_max=0.01 m^2  del_S_orifice_area_TLU=[0, .003, .006, .009, .012, .015] m  orifice_area_TLU=[1e-10, 2e-05, 4e-05, 6e-05, 8e-05, .0001] m^2  Cd=0.8  leakage_fraction=1e-6  smoothing_factor=0.01  B_lam=0.999  area=0.015 m^2  S_max_PA=-0.01 m  del_S_max_PA=0.005 m  Cv_max_PA=4  del_S_Cv_TLU_PA=[0, .001, .002, .003, .004, .005] m  Cv_TLU_PA=[1e-06, .8, 1.6, 2.4, 3.2, 4]  xT_Cv_PA=0.7  Kv_max_PA=3.6  del_S_Kv_TLU_PA=[0, .001, .002, .003, .004, .005] m  Kv_TLU_PA=[1e-06, .72, 1.44, 2.16, 2.88, 3.6]  xT_Kv_PA=0.7  C_max_PA=12 l/(bar*s)  B_crit_linear_PA=0.3  del_S_C_TLU_PA=[0, .001, .002, .003, .004, .005] m  C_TLU_PA=[1e-05, 2.4, 4.8, 7.2, 9.6, 12] l/(bar*s)  B_crit_TLU_PA=0.3 * ones(1, 6)  m_PA=0.5  T_ref_C_PA=293.15 K  rho_ref_C_PA=1.185 kg/m^3  orifice_area_max_PA=1e-4 m^2  del_S_orifice_area_TLU_PA=[0, .001, .002, .003, .004, .005] m  orifice_area_TLU_PA=[1e-10, 2e-05, 4e-05, 6e-05, 8e-05, .0001] m^2  S_max_AT=0.01 m  del_S_max_AT=0.005 m  Cv_max_AT=4  del_S_Cv_TLU_AT=[0, .001, .002, .003, .004, .005] m  Cv_TLU_AT=[1e-06, .8, 1.6, 2.4, 3.2, 4]  xT_Cv_AT=0.7  Kv_max_AT=3.6  del_S_Kv_TLU_AT=[0, .001, .002, .003, .004, .005] m  Kv_TLU_AT=[1e-06, .72, 1.44, 2.16, 2.88, 3.6]  xT_Kv_AT=0.7  C_max_AT=12 l/(bar*s)  B_crit_linear_AT=0.3  del_S_C_TLU_AT=[0, .001, .002, .003, .004, .005] m  C_TLU_AT=[1e-05, 2.4, 4.8, 7.2, 9.6, 12] l/(bar*s)  B_crit_TLU_AT=0.3 * ones(1, 6)  m_AT=0.5  T_ref_C_AT=293.15 K  rho_ref_C_AT=1.185 kg/m^3  orifice_area_max_AT=1e-4 m^2  del_S_orifice_area_TLU_AT=[0, .001, .002, .003, .004, .005] m  orifice_area_TLU_AT=[1e-10, 2e-05, 4e-05, 6e-05, 8e-05, .0001] m^2  S_max_PT=4.5e-3 m  del_S_max_PT=0.005 m  Cv_max_PT=4  del_S_Cv_TLU_PT=[0, .001, .002, .003, .004, .005] m  Cv_TLU_PT=[1e-06, .8, 1.6, 2.4, 3.2, 4]  xT_Cv_PT=0.7  Kv_max_PT=3.6  del_S_Kv_TLU_PT=[0, .001, .002, .003, .004, .005] m  Kv_TLU_PT=[1e-06, .72, 1.44, 2.16, 2.88, 3.6]  xT_Kv_PT=0.7  C_max_PT=12 l/(bar*s)  B_crit_linear_PT=0.3  del_S_C_TLU_PT=[0, .001, .002, .003, .004, .005] m  C_TLU_PT=[1e-05, 2.4, 4.8, 7.2, 9.6, 12] l/(bar*s)  B_crit_TLU_PT=0.3 * ones(1, 6)  m_PT=0.5  T_ref_C_PT=293.15 K  rho_ref_C_PT=1.185 kg/m^3  orifice_area_max_PT=1e-4 m^2  del_S_orifice_area_TLU_PT=[0, .001, .002, .003, .004, .005] m  orifice_area_TLU_PT=[1e-10, 2e-05, 4e-05, 6e-05, 8e-05, .0001] m^2
      settings: InternalSimscapePortConfiguration="{\"Bottom\":[{\"id\":\"P\",\"label\":\"P\",\"type\":\"foundation.moist_air.moist_air\"},{\"id\":\"T\",\"label\":\"T\",\"type\":\"foundation.moist_air.moist_air\"}],\"Left\":[{\"id\":\"S\",\"label\":\"S\",\"type\":\"input\"}],\"Right\":[],\"Top\":[{\"id\":\"A\",\"label\":\"A\",\"type\":\"foundation.moist_air.moist_air\"}]}"
  Flow Rate Sensor (MA) : fl_lib/Moist Air/Sensors/Flow Rate Sensor (MA)  mass_flow_measure=true  volumetric_flow_measure=false  volumetric_flow_conditions=foundation.enum.volumetric_flow_conditions.actual  p_std=0.101325 MPa  T_std=20 degC  RH_std=0.65  energy_flow_measure=true  vapor_flow_measure=false  gas_flow_measure=false  droplets_flow_measure=false
      settings: InternalSimscapePortConfiguration="{\"Bottom\":[{\"id\":\"PHI\",\"label\":\"φ\",\"type\":\"output\"}],\"Left\":[{\"id\":\"A\",\"label\":\"A\",\"type\":\"foundation.moist_air.moist_air\"}],\"Right\":[{\"id\":\"B\",\"label\":\"B\",\"type\":\"foundation.moist_air.moist_air\"},{\"id\":\"M\",\"label\":\"M\",\"type\":\"output\"}],\"Top\":[]}"
  Flow Rate Sensor (MA)2 : fl_lib/Moist Air/Sensors/Flow Rate Sensor (MA)  mass_flow_measure=true  volumetric_flow_measure=false  volumetric_flow_conditions=foundation.enum.volumetric_flow_conditions.actual  p_std=0.101325 MPa  T_std=20 degC  RH_std=0.65  energy_flow_measure=true  vapor_flow_measure=false  gas_flow_measure=false  droplets_flow_measure=false
      settings: InternalSimscapePortConfiguration="{\"Bottom\":[{\"id\":\"PHI\",\"label\":\"φ\",\"type\":\"output\"}],\"Left\":[{\"id\":\"A\",\"label\":\"A\",\"type\":\"foundation.moist_air.moist_air\"}],\"Right\":[{\"id\":\"B\",\"label\":\"B\",\"type\":\"foundation.moist_air.moist_air\"},{\"id\":\"M\",\"label\":\"M\",\"type\":\"output\"}],\"Top\":[]}"
  PS-Simulink Converter12 : nesl_utility/PS-Simulink Converter  PhysicalDomain=network_engine_domain  SubClassName=ps_output  LeftPortType=input  RightPortType=output  PseudoPeriodic=off  Frequencies=[]  VectorFormat=inherit  Unit=inherit  AffineConversion=off
  PS-Simulink Converter7 : nesl_utility/PS-Simulink Converter  PhysicalDomain=network_engine_domain  SubClassName=ps_output  LeftPortType=input  RightPortType=output  PseudoPeriodic=off  Frequencies=[]  VectorFormat=inherit  Unit=inherit  AffineConversion=off
  Simulink-PS Converter8 : nesl_utility/Simulink-PS Converter  PhysicalDomain=network_engine_domain  SubClassName=ps_input  LeftPortType=input  RightPortType=output  PseudoPeriodic=off  Frequencies=[]  NoiseDistribution=none  NoiseParameters=[]  Unit=1  AffineConversion=off  FilteringAndDerivatives=provide  SimscapeFilterOrder=1  InputFilterTimeConstant=0.001  UdotUserProvided=0
  A : PMIOPort  Side=Left
  B2 : PMIOPort  Port=2  Side=Right
  B1 : PMIOPort  Port=3  Side=Right
  tag scope: f_MA_Evap=global, f_MA_WaterCoil=global
  wires:
  PS-Simulink Converter7/1 -> [f_MA_Evap]
  PS-Simulink Converter12/1 -> [f_MA_WaterCoil]
  [V_Discharge] -> Simulink-PS Converter8/1
  connections:
  Flow Rate Sensor (MA)2/RConn2 -- PS-Simulink Converter12/LConn1
  Flow Rate Sensor (MA)/RConn2 -- PS-Simulink Converter7/LConn1
  Simulink-PS Converter8/RConn1 -- 3-Way Directional Valve (MA)/LConn1
  A/RConn1 -- 3-Way Directional Valve (MA)/LConn2
  Flow Rate Sensor (MA)/RConn1 -- B1/RConn1
  Flow Rate Sensor (MA)2/RConn1 -- B2/RConn1
  Flow Rate Sensor (MA)2/LConn1 -- 3-Way Directional Valve (MA)/RConn1
  Flow Rate Sensor (MA)/LConn1 -- 3-Way Directional Valve (MA)/RConn2

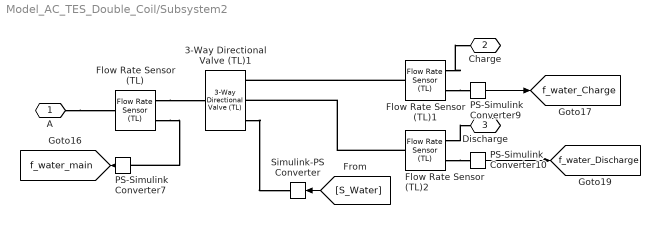
== system Model_AC_TES_Double_Coil/Subsystem2 ==
  3-Way Directional Valve (TL)1 : SimscapeFluids_lib/Thermal Liquid/Valves & Orifices/Directional Control Valves/3-Way Directional Valve (TL)  open_orifices_pos=fluids.thermal_liquid.valves.directional_control_valves.enum.OpenOrifices3Way.PA  open_orifices_neg=fluids.thermal_liquid.valves.directional_control_valves.enum.OpenOrifices3Way.AT  area_spec=fluids.thermal_liquid.valves.directional_control_valves.enum.area_spec.identical  valve_spec=fluids.thermal_liquid.valves.directional_control_valves.enum.ValveSpec.Linear  del_S_max=0.01 m  area_max=0.01 m^2  del_S_TLU=[0, .00125, .0025, .00375, .005] m  valve_area_TLU=[1e-10, 1e-05, 4e-05, 8e-05, .0001] m^2  del_S_flow_TLU=[0, .00125, .0025, .00375, .005] m  p_diff_TLU=[-.1, .3, .5, .7] MPa  vol_flow_TLU=[-9.05e-10, 1.57e-09, 2.02e-09, 2.39e-09; -9.05e-05, .000157, .000202, .000239; -.000362, .000627, .00081, .000958; -.000724, .00125, .00162, .00192; -.000905, .00156, .002, .00239] m^3/s  mdot_TLU=1e3 * [-9.05e-10, 1.57e-09, 2.02e-09, 2.39e-09; -9.05e-05, .000157, .000202, .000239; -.000362, .000627, .00081, .000958; -.000724, .00125, .00162, .00192; -.000905, .00156, .002, .00239] kg/s  T_ref_in=293.15 K  p_ref_in=0.101325 MPa  area_leak=1e-10 m^2  Cd=0.8  Re_c=150  smoothing_factor=0.01  pressure_recovery=false  area=0.015 m^2  S_max_PA=0.01 m  del_S_max_PA=0.005 m  area_max_PA=1e-4 m^2  del_S_TLU_PA=[0, .00125, .0025, .00375, .005] m  valve_area_TLU_PA=[1e-10, 1e-05, 4e-05, 8e-05, .0001] m^2  del_S_flow_TLU_PA=[0, .00125, .0025, .00375, .005] m  p_diff_TLU_PA=[-.1, .3, .5, .7] MPa  vol_flow_TLU_PA=[-9.05e-10, 1.57e-09, 2.02e-09, 2.39e-09; -9.05e-05, .000157, .000202, .000239; -.000362, .000627, .00081, .000958; -.000724, .00125, .00162, .00192; -.000905, .00156, .002, .00239] m^3/s  mdot_TLU_PA=1e3 * [-9.05e-10, 1.57e-09, 2.02e-09, 2.39e-09; -9.05e-05, .000157, .000202, .000239; -.000362, .000627, .00081, .000958; -.000724, .00125, .00162, .00192; -.000905, .00156, .002, .00239] kg/s  S_max_AT=-0.01 m  del_S_max_AT=0.005 m  area_max_AT=1e-4 m^2  del_S_TLU_AT=[0, .00125, .0025, .00375, .005] m  valve_area_TLU_AT=[1e-10, 1e-05, 4e-05, 8e-05, .0001] m^2  del_S_flow_TLU_AT=[0, .00125, .0025, .00375, .005] m  p_diff_TLU_AT=[-.1, .3, .5, .7] MPa  vol_flow_TLU_AT=[-9.05e-10, 1.57e-09, 2.02e-09, 2.39e-09; -9.05e-05, .000157, .000202, .000239; -.000362, .000627, .00081, .000958; -.000724, .00125, .00162, .00192; -.000905, .00156, .002, .00239] m^3/s  mdot_TLU_AT=1e3 * [-9.05e-10, 1.57e-09, 2.02e-09, 2.39e-09; -9.05e-05, .000157, .000202, .000239; -.000362, .000627, .00081, .000958; -.000724, .00125, .00162, .00192; -.000905, .00156, .002, .00239] kg/s  S_max_PT=4.5e-3 m  del_S_max_PT=0.005 m  area_max_PT=1e-4 m^2  del_S_TLU_PT=[0, .00125, .0025, .00375, .005] m  valve_area_TLU_PT=[1e-10, 1e-05, 4e-05, 8e-05, .0001] m^2  del_S_flow_TLU_PT=[0, .00125, .0025, .00375, .005] m  p_diff_TLU_PT=[-.1, .3, .5, .7] MPa  vol_flow_TLU_PT=[-9.05e-10, 1.57e-09, 2.02e-09, 2.39e-09; -9.05e-05, .000157, .000202, .000239; -.000362, .000627, .00081, .000958; -.000724, .00125, .00162, .00192; -.000905, .00156, .002, .00239] m^3/s  mdot_TLU_PT=1e3 * [-9.05e-10, 1.57e-09, 2.02e-09, 2.39e-09; -9.05e-05, .000157, .000202, .000239; -.000362, .000627, .00081, .000958; -.000724, .00125, .00162, .00192; -.000905, .00156, .002, .00239] kg/s
      settings: InternalSimscapePortConfiguration="{\"Bottom\":[],\"Left\":[{\"id\":\"A\",\"label\":\"A\",\"type\":\"foundation.thermal_liquid.thermal_liquid\"}],\"Right\":[{\"id\":\"S\",\"label\":\"S\",\"type\":\"input\"},{\"id\":\"P\",\"label\":\"P\",\"type\":\"foundation.thermal_liquid.thermal_liquid\"},{\"id\":\"T\",\"label\":\"T\",\"type\":\"foundation.thermal_liquid.thermal_liquid\"}],\"Top\":[]}"
  Flow Rate Sensor (TL) : fl_lib/Thermal Liquid/Sensors/Flow Rate Sensor (TL)  mass_flow_measure=true  volumetric_flow_measure=false  energy_flow_measure=false
      settings: InternalSimscapePortConfiguration="{\"Bottom\":[],\"Left\":[{\"id\":\"A\",\"label\":\"A\",\"type\":\"foundation.thermal_liquid.thermal_liquid\"}],\"Right\":[{\"id\":\"B\",\"label\":\"B\",\"type\":\"foundation.thermal_liquid.thermal_liquid\"},{\"id\":\"M\",\"label\":\"M\",\"type\":\"output\"}],\"Top\":[]}"
  Flow Rate Sensor (TL)1 : fl_lib/Thermal Liquid/Sensors/Flow Rate Sensor (TL)  mass_flow_measure=true  volumetric_flow_measure=false  energy_flow_measure=false
      settings: InternalSimscapePortConfiguration="{\"Bottom\":[],\"Left\":[{\"id\":\"A\",\"label\":\"A\",\"type\":\"foundation.thermal_liquid.thermal_liquid\"}],\"Right\":[{\"id\":\"B\",\"label\":\"B\",\"type\":\"foundation.thermal_liquid.thermal_liquid\"},{\"id\":\"M\",\"label\":\"M\",\"type\":\"output\"}],\"Top\":[]}"
  Flow Rate Sensor (TL)2 : fl_lib/Thermal Liquid/Sensors/Flow Rate Sensor (TL)  mass_flow_measure=true  volumetric_flow_measure=false  energy_flow_measure=false
      settings: InternalSimscapePortConfiguration="{\"Bottom\":[],\"Left\":[{\"id\":\"A\",\"label\":\"A\",\"type\":\"foundation.thermal_liquid.thermal_liquid\"}],\"Right\":[{\"id\":\"B\",\"label\":\"B\",\"type\":\"foundation.thermal_liquid.thermal_liquid\"},{\"id\":\"M\",\"label\":\"M\",\"type\":\"output\"}],\"Top\":[]}"
  PS-Simulink Converter10 : nesl_utility/PS-Simulink Converter  PhysicalDomain=network_engine_domain  SubClassName=ps_output  LeftPortType=input  RightPortType=output  PseudoPeriodic=off  Frequencies=[]  VectorFormat=inherit  Unit=1  AffineConversion=off
  PS-Simulink Converter7 : nesl_utility/PS-Simulink Converter  PhysicalDomain=network_engine_domain  SubClassName=ps_output  LeftPortType=input  RightPortType=output  PseudoPeriodic=off  Frequencies=[]  VectorFormat=inherit  Unit=1  AffineConversion=off
  PS-Simulink Converter9 : nesl_utility/PS-Simulink Converter  PhysicalDomain=network_engine_domain  SubClassName=ps_output  LeftPortType=input  RightPortType=output  PseudoPeriodic=off  Frequencies=[]  VectorFormat=inherit  Unit=1  AffineConversion=off
  Simulink-PS Converter : nesl_utility/Simulink-PS Converter  PhysicalDomain=network_engine_domain  SubClassName=ps_input  LeftPortType=input  RightPortType=output  PseudoPeriodic=off  Frequencies=[]  NoiseDistribution=none  NoiseParameters=[]  Unit=1  AffineConversion=off  FilteringAndDerivatives=provide  SimscapeFilterOrder=1  InputFilterTimeConstant=0.001  UdotUserProvided=0
  A : PMIOPort  Side=Left
  Charge : PMIOPort  Port=2  Side=Right
  Discharge : PMIOPort  Port=3  Side=Right
  tag scope: f_water_Charge=global, f_water_Discharge=global, f_water_main=global
  wires:
  PS-Simulink Converter9/1 -> [f_water_Charge]
  PS-Simulink Converter10/1 -> [f_water_Discharge]
  PS-Simulink Converter7/1 -> [f_water_main]
  [S_Water] -> Simulink-PS Converter/1
  connections:
  Flow Rate Sensor (TL)/RConn2 -- PS-Simulink Converter7/LConn1
  Flow Rate Sensor (TL)/RConn1 -- 3-Way Directional Valve (TL)1/LConn1
  3-Way Directional Valve (TL)1/RConn1 -- Simulink-PS Converter/RConn1
  Flow Rate Sensor (TL)1/RConn2 -- PS-Simulink Converter9/LConn1
  Flow Rate Sensor (TL)2/RConn2 -- PS-Simulink Converter10/LConn1
  Flow Rate Sensor (TL)2/LConn1 -- 3-Way Directional Valve (TL)1/RConn2
  Flow Rate Sensor (TL)2/RConn1 -- Discharge/RConn1
  Flow Rate Sensor (TL)1/RConn1 -- Charge/RConn1
  A/RConn1 -- Flow Rate Sensor (TL)/LConn1
  Flow Rate Sensor (TL)1/LConn1 -- 3-Way Directional Valve (TL)1/RConn3

== system Model_AC_TES_Double_Coil/Subsystem3 ==
  Ideal Angular Velocity Source : fl_lib/Mechanical/Mechanical Sources/Ideal Angular Velocity Source
  Mechanical Rotational Reference : fl_lib/Mechanical/Rotational Elements/Mechanical Rotational Reference
  PS Gain : fl_lib/Physical Signals/Functions/PS Gain  gain=950 rpm
  Simulink-PS Converter2 : nesl_utility/Simulink-PS Converter  PhysicalDomain=network_engine_domain  SubClassName=ps_input  LeftPortType=input  RightPortType=output  PseudoPeriodic=off  Frequencies=[]  NoiseDistribution=none  NoiseParameters=[]  Unit=1  AffineConversion=off  FilteringAndDerivatives=provide  SimscapeFilterOrder=1  InputFilterTimeConstant=0.001  UdotUserProvided=0
  R : PMIOPort  Side=Left
  C : PMIOPort  Port=2  Side=Right
  wires:
  [on_off_Conpsr] -> Simulink-PS Converter2/1
  connections:
  Ideal Angular Velocity Source/RConn2 -- C/RConn1
  Simulink-PS Converter2/RConn1 -- PS Gain/LConn1
  Ideal Angular Velocity Source/LConn1 -- Mechanical Rotational Reference/LConn1 -- R/RConn1
  PS Gain/RConn1 -- Ideal Angular Velocity Source/RConn1

== stateflow chart Model_AC_TES_Double_Coil/Chart2 ==
  state Charge
    entry :Evap = 0;Comp=1;Cond=1;
    Pump = 1;
    V_R32 = -1;
    V_main = -1;
    V_discharge =1;
  state ChangValve1
    entry :Evap = 0;Comp=0;Cond=0;
    Pump = 1;
    V_R32 = 1;
    V_main = -1;
    V_discharge =1;
  state Off
    entry :Evap = 0;Comp=0;Cond=0;
    Pump = 0;
    V_R32 = 1;
    V_main = -1;
    V_discharge =1;
  state ChangeValve2
    entry :Evap = 0;Comp=0;Cond=0;
    Pump = 0;
    V_R32 = 1;
    V_main = 1;
    V_discharge =-1;
  state Discharge
    entry :Evap = 0.3;Comp=0;Cond=0;
    Pump = 0.5;
  state AC
    entry :Evap = 0.9;Comp=1;Cond=1;
    Pump = 0;
    V_R32 = 1;
    V_main = 1;
    V_discharge =1;
  (default) -> Charge
  Charge -> ChangValve1 : [T_Tank <=8]
  ChangValve1 -> Off : [after(60,sec)]
  Off -> ChangeValve2 : [after(60,sec)]
  ChangeValve2 -> Discharge : [after(5,sec)]
  Discharge -> AC : [T_Tank>18]
  data: T_Tank input; Comp output; Cond output; Evap output; Pump output; V_R32 output; T_Room input; V_discharge output; V_main output
